simulink model "EPS_orbit_v4a"  (R2023b)
settings: Solver=FixedStepAuto  StartTime=0.0  StopTime=tsimulation  FixedStep=delta_t  RelTol=1e-3
undefined symbols (not defined in the file or in its folder): att, date, juliandate, MODE, SP
libraries: dspmathops x17, vrlib x12, aerolibutil x10, sharedtransform x8, sharedutil x4
(part 2 of 2)

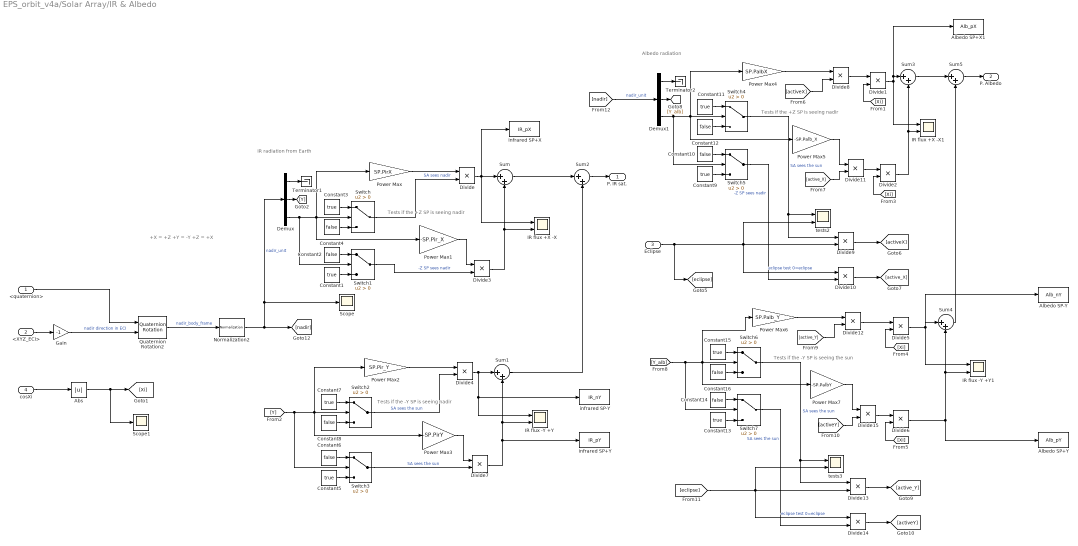
== system EPS_orbit_v4a/Solar Array/IR & Albedo ==
  note: Albedo radiation
  note: IR radiation from Earth
  note: +X = +Z
      | +Y = -Y
      | +Z = +X
  note: Tests if the -Y SP is seeing nadir
  note: Tests if the +Z SP is seeing nadir
  note: Tests if the +Z SP is seeing nadir
  note: Tests if the -Y SP is seeing the sun
  <quaternion> : Inport
  <XYZ_ECI> : Inport  Port=2
  Eclipse : Inport  Port=3
  cosXi : Inport  Port=4
  Abs : Abs  SaturateOnIntegerOverflow=off
  Albedo SP+X1 : ToWorkspace  VariableName=Alb_pX  SaveFormat=Timeseries  SampleTime=1
      settings: Save2DSignal=2-D array (concatenate along first dimension)
  Albedo SP+Y : ToWorkspace  VariableName=Alb_pY  SaveFormat=Timeseries  SampleTime=1
      settings: Save2DSignal=2-D array (concatenate along first dimension)
  Albedo SP-Y : ToWorkspace  VariableName=Alb_nY  SaveFormat=Timeseries  SampleTime=1
      settings: Save2DSignal=2-D array (concatenate along first dimension)
  Constant{1,3,5,7,9,11,13,15} (8 alike) : Constant  Value=true
  Constant{2,4,6,8,10,12,14,16} (8 alike) : Constant  Value=false
  Demux : Demux  Outputs=3
  Demux1 : Demux  Outputs=3
  Divide{,1..15} (16 alike) : Product  Inputs=**
  Gain : Gain  Gain=-1
  IR flux +X -X : Scope  NumInputPorts=2
  IR flux +X -X1 : Scope  NumInputPorts=2
  IR flux -Y +Y : Scope  NumInputPorts=2
  IR flux -Y +Y1 : Scope  NumInputPorts=2
  Normalization2 : dspmathops/Normalization  NormType=2-norm  Bias=1e-10  NormOver=Each column  Dimension=1  roundingMode=Floor  overflowMode=off  accumDataTypeStr=Inherit: Same as product output  accumLastDataTypeStr=Inherit: Same as product output  outputDataTypeStr=Inherit: Same as product output  outputMin=[]  outputMax=[]  outputLastDataTypeStr=Inherit: Same as product output
  Power Max : Gain  Gain=SP.PirX
  Power Max1 : Gain  Gain=-SP.Pir_X
  Power Max2 : Gain  Gain=SP.Pir_Y
  Power Max3 : Gain  Gain=-SP.PirY
  Power Max4 : Gain  Gain=SP.PalbX
  Power Max5 : Gain  Gain=-SP.Palb_X
  Power Max6 : Gain  Gain=SP.Palb_Y
  Power Max7 : Gain  Gain=-SP.PalbY
  Quaternion Rotation2 : aerolibutil/Quaternion Rotation
  Scope : Scope
  Scope1 : Scope
  Sum{,1..5} (6 alike) : Sum  Inputs=|++
  Switch{,1..7} (8 alike) : Switch  Criteria=u2 > Threshold  SaturateOnIntegerOverflow=off  InputSameDT=off
  Terminator1 : Terminator
  Terminator2 : Terminator
  infrared SP+X : ToWorkspace  VariableName=IR_pX  SaveFormat=Timeseries  SampleTime=1
      settings: Save2DSignal=2-D array (concatenate along first dimension)
  infrared SP+Y : ToWorkspace  VariableName=IR_pY  SaveFormat=Timeseries  SampleTime=1
      settings: Save2DSignal=2-D array (concatenate along first dimension)
  infrared SP-Y : ToWorkspace  VariableName=IR_nY  SaveFormat=Timeseries  SampleTime=1
      settings: Save2DSignal=2-D array (concatenate along first dimension)
  tests2 : Scope  NumInputPorts=2
  tests3 : Scope  NumInputPorts=2
  P. IR sat. : Outport
  P. Albedo : Outport  Port=2
  wires:
  Gain/1 -> Quaternion Rotation2/2  "nadir direction in ECI"
  <XYZ_ECI>/1 -> Gain/1
  Quaternion Rotation2/1 -> Normalization2/1  "nadir_body_frame"
  <quaternion>/1 -> Quaternion Rotation2/1
  Sum2/1 -> P. IR sat./1
  Switch3/1 -> Divide7/2  "SA sees the sun"
  Divide7/1 -> infrared SP+Y/1, IR flux -Y +Y/2, Sum1/2
  Power Max2/1 -> Divide4/1
  Divide4/1 -> infrared SP-Y/1, IR flux -Y +Y/1, Sum1/1
  Power Max3/1 -> Divide7/1
  Constant4/1 -> Switch/3
  Constant6/1 -> Switch3/1
  Constant5/1 -> Switch3/3
  Power Max/1 -> Divide/1
  Switch2/1 -> Divide4/2  "SA sees the sun"
  Demux/1 -> Terminator1/1
  Constant8/1 -> Switch2/3
  Divide3/1 -> Sum/2, IR flux +X -X/2
  Sum1/1 -> Sum2/2
  Power Max1/1 -> Divide3/1
  Constant7/1 -> Switch2/1
  Constant3/1 -> Switch/1
  Sum/1 -> Sum2/1
  [Y] -> Switch2/2, Power Max3/1, Power Max2/1, Switch3/2
  Demux/3 -> Switch1/2, Power Max1/1, Power Max/1, Switch/2
  Constant1/1 -> Switch1/3
  Demux/2 -> [Y]
  Switch/1 -> Divide/2  "SA sees nadir"
  Constant2/1 -> Switch1/1
  Normalization2/1 -> Scope/1, Demux/1, [nadir]  "nadir_unit"
  Divide/1 -> infrared SP+X/1, IR flux +X -X/1, Sum/1
  Switch1/1 -> Divide3/2  "-Z SP sees nadir"
  Switch5/1 -> Divide10/2  "-Z SP sees nadir"
  Divide8/1 -> Divide1/1
  Switch4/1 -> Divide9/1, tests2/1  "SA sees the sun"
  Divide10/1 -> [active_X]
  [Y_alb] -> Switch7/2, Power Max7/1, Power Max6/1, Switch6/2
  [activeX] -> Divide8/2
  Divide13/1 -> [active_Y]
  Sum3/1 -> Sum5/1
  Constant11/1 -> Switch4/1
  Constant15/1 -> Switch6/1
  Demux1/3 -> Switch5/2, Power Max5/1, Power Max4/1, Switch4/2
  Constant16/1 -> Switch6/3
  Demux1/2 -> [Y_alb]
  Power Max4/1 -> Divide8/1
  Divide14/1 -> [activeY]
  Demux1/1 -> Terminator2/1
  Switch6/1 -> Divide13/1, tests3/1  "SA sees the sun"
  Divide11/1 -> Divide2/1
  Constant9/1 -> Switch5/3
  Constant12/1 -> Switch4/3
  Constant14/1 -> Switch7/1
  [active_X] -> Divide11/2
  [active_Y] -> Divide12/2
  Constant10/1 -> Switch5/1
  [activeY] -> Divide15/2
  Power Max7/1 -> Divide15/1
  [eclipse] -> Divide14/1, tests3/2, Divide13/2  "eclipse test 0=eclipse"
  Switch7/1 -> Divide14/2  "SA sees the sun"
  Divide9/1 -> [activeX]
  Divide6/1 -> IR flux -Y +Y1/2, Sum4/2, Albedo SP+Y/1
  Divide12/1 -> Divide5/1
  Power Max5/1 -> Divide11/1
  Constant13/1 -> Switch7/3
  Power Max6/1 -> Divide12/1
  Sum4/1 -> Sum5/2
  Sum5/1 -> P. Albedo/1
  Eclipse/1 -> Divide10/1, tests2/2, Divide9/2, [eclipse]  "eclipse test 0=eclipse"
  [nadir] -> Demux1/1  "nadir_unit"
  cosXi/1 -> Abs/1
  Abs/1 -> [Xi], Scope1/1
  Divide1/1 -> Albedo SP+X1/1, Sum3/1, IR flux +X -X1/1
  [Xi] -> Divide1/2
  [Xi] -> Divide2/2
  Divide2/1 -> IR flux +X -X1/2, Sum3/2
  [Xi] -> Divide5/2
  Divide15/1 -> Divide6/1
  [Xi] -> Divide6/2
  Divide5/1 -> Albedo SP-Y/1, IR flux -Y +Y1/1, Sum4/1

== matlab function EPS_orbit_v4a/Subsystem/JD to UTC ==
  data: JD input; Time_UTC output
function Time_UTC = fcn(JD)
    coder.extrinsic('datetime','datevec');
    Time_UTC = [0,0,0,0,0,0];
Time_UTC =  datevec(datetime(JD,'convertfrom','juliandate'));
